simulink model "MSD2_RLS"  (R2019a)
settings: Solver=ode45  StartTime=t0  StopTime=tend  MaxStep=maxstep  RelTol=tol  AbsTol=tol
values from neighbouring files (symbols this model uses):
  d = 0.5    [SimMSD2_RLS.m]
  dx10 = 0    [SimMSD2_RLS.m]
  dx20 = 0    [SimMSD2_RLS.m]
  Fmag = 3    [SimMSD2_RLS.m]
  lambda = 0.99    [SimMSD2_RLS.m]
  P0 = 1e8 * eye(n_theta)    [SimMSD2_RLS.m]
  params_true = [m1 m2 k1 k2 c1 c2 b].'    [SimMSD2_RLS.m]
  T = 0.01    [SimMSD2_RLS.m]
  tend = 30    [SimMSD2_RLS.m]
  theta0 = genTheta(params0)    [SimMSD2_RLS.m]
  x10 = 0    [SimMSD2_RLS.m]
  x20 = x10    (= 0)    [SimMSD2_RLS.m]
  z0 = [x10 x20 dx10 dx20].'    [SimMSD2_RLS.m]
settings Model: Creator=bednarse  LastModifiedBy=bednarse

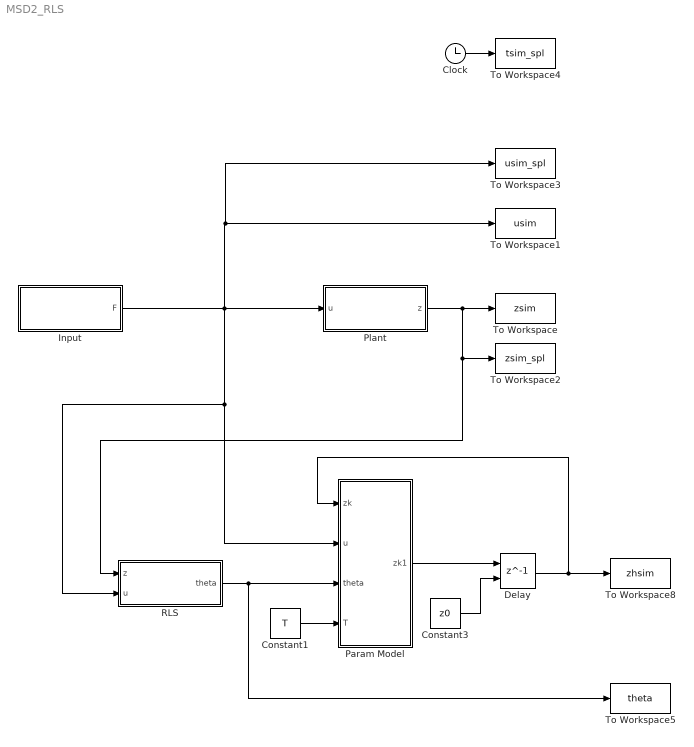
== system MSD2_RLS ==
  Clock : Clock
  Constant1 : Constant  Value=T
  Constant3 : Constant  Value=z0
  Delay : Delay  DelayLength=1  InitialConditionSource=Input port
      settings: InputPortMap=u0,p4
  Input : Subsystem
  Param Model : MATLAB Function  TreatAsAtomicUnit=on  SystemSampleTime=T
  Plant : Subsystem
  RLS : Subsystem
  To Workspace : ToWorkspace  VariableName=zsim  SampleTime=-1
  To Workspace1 : ToWorkspace  VariableName=usim  SampleTime=-1
  To Workspace2 : ToWorkspace  VariableName=zsim_spl  SampleTime=T
  To Workspace3 : ToWorkspace  VariableName=usim_spl  SampleTime=T
  To Workspace4 : ToWorkspace  VariableName=tsim_spl  SampleTime=T
  To Workspace5 : ToWorkspace  VariableName=theta  SampleTime=-1
  To Workspace8 : ToWorkspace  VariableName=zhsim  SampleTime=T
  wires:
  Plant/1(z) -> RLS/1(z), To Workspace2/1, To Workspace/1
  Clock/1 -> To Workspace4/1
  Param Model/1(zk1) -> Delay/1
  Constant1/1 -> Param Model/4(T)
  Constant3/1 -> Delay/2
  Delay/1 -> Param Model/1(zk), To Workspace8/1
  Input/1(F) -> Param Model/2(u), RLS/2(u), To Workspace3/1, To Workspace1/1, Plant/1(u)
  RLS/1(theta) -> To Workspace5/1, Param Model/3(theta)

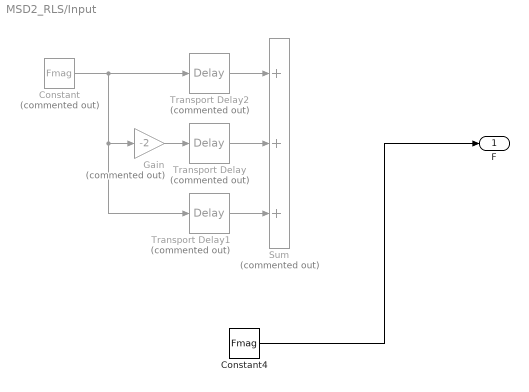
== system MSD2_RLS/Input ==
  Constant : Constant  Commented=on  Value=Fmag
  Constant4 : Constant  Value=Fmag
  Gain : Gain  Commented=on  Gain=-2
  Sum : Sum  Commented=on  Inputs=+++
  Transport Delay : TransportDelay  Commented=on  DelayTime=2*d  BufferSize=2048
  Transport Delay1 : TransportDelay  Commented=on  DelayTime=3*d  BufferSize=4096
  Transport Delay2 : TransportDelay  Commented=on  DelayTime=d
  F : Outport
  wires:
  Gain/1 -> Transport Delay/1
  Transport Delay1/1 -> Sum/3
  Transport Delay2/1 -> Sum/1
  Transport Delay/1 -> Sum/2
  Constant/1 -> Transport Delay1/1, Gain/1, Transport Delay2/1
  Constant4/1 -> F/1

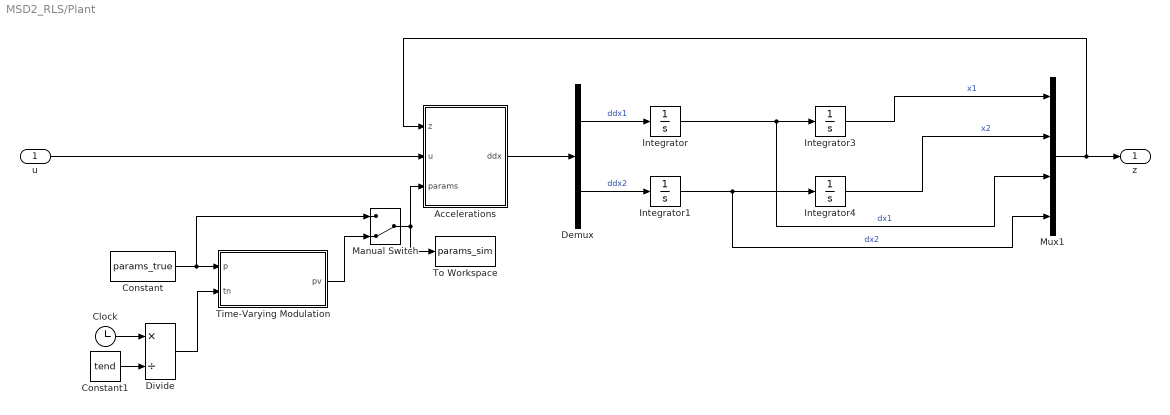
== system MSD2_RLS/Plant ==
  u : Inport
  Accelerations : MATLAB Function  TreatAsAtomicUnit=on
  Clock : Clock
  Constant : Constant  Value=params_true
  Constant1 : Constant  Value=tend
  Demux : Demux  Outputs=2
  Divide : Product  Inputs=*/
  Integrator : Integrator  InitialCondition=dx10
  Integrator1 : Integrator  InitialCondition=dx20
  Integrator3 : Integrator  InitialCondition=x10
  Integrator4 : Integrator  InitialCondition=x20
  Manual Switch : ManualSwitch  CurrentSetting=0
  Mux1 : Mux
  Time-Varying Modulation : MATLAB Function  TreatAsAtomicUnit=on
  To Workspace : ToWorkspace  VariableName=params_sim  SampleTime=-1
  z : Outport
  wires:
  Integrator3/1 -> Mux1/1  "x1"
  Integrator4/1 -> Mux1/2  "x2"
  Demux/2 -> Integrator1/1  "ddx2"
  Accelerations/1(ddx) -> Demux/1
  Demux/1 -> Integrator/1  "ddx1"
  Integrator/1 -> Mux1/3, Integrator3/1  "dx1"
  Integrator1/1 -> Mux1/4, Integrator4/1  "dx2"
  u/1 -> Accelerations/2(u)
  Mux1/1 -> Accelerations/1(z), z/1
  Clock/1 -> Divide/1
  Constant1/1 -> Divide/2
  Time-Varying Modulation/1(pv) -> Manual Switch/2
  Constant/1 -> Manual Switch/1, Time-Varying Modulation/1(p)
  Divide/1 -> Time-Varying Modulation/2(tn)
  Manual Switch/1 -> Accelerations/3(params), To Workspace/1

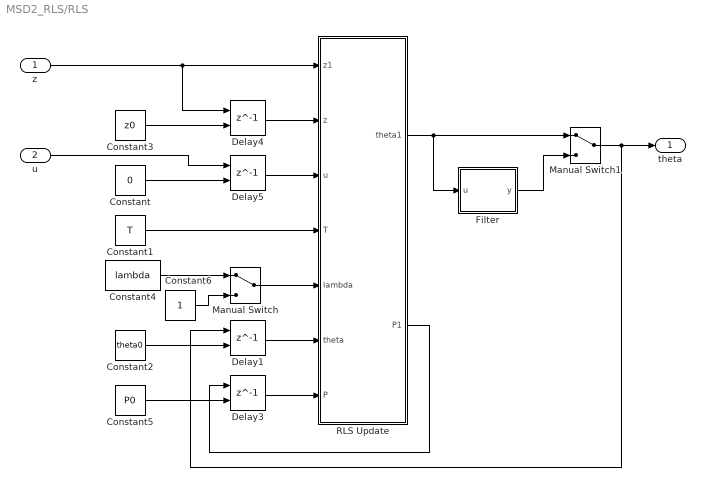
== system MSD2_RLS/RLS ==
  z : Inport
  u : Inport  Port=2
  Constant : Constant  Value=0
  Constant1 : Constant  Value=T
  Constant2 : Constant  Value=theta0
  Constant3 : Constant  Value=z0
  Constant4 : Constant  Value=lambda
  Constant5 : Constant  Value=P0
  Constant6 : Constant
  Delay{1,3..5} (4 alike) : Delay  DelayLength=1  InitialConditionSource=Input port
      settings: InputPortMap=u0,p4
  Filter : Subsystem
  Manual Switch : ManualSwitch
  Manual Switch1 : ManualSwitch
  RLS Update : MATLAB Function  TreatAsAtomicUnit=on  SystemSampleTime=T
  theta : Outport
  wires:
  Constant/1 -> Delay5/2
  Constant3/1 -> Delay4/2
  Constant5/1 -> Delay3/2
  Constant1/1 -> RLS Update/4(T)
  Constant2/1 -> Delay1/2
  Delay5/1 -> RLS Update/3(u)
  Delay4/1 -> RLS Update/2(z)
  Delay3/1 -> RLS Update/7(P)
  Delay1/1 -> RLS Update/6(theta)
  RLS Update/2(P1) -> Delay3/1
  u/1 -> Delay5/1
  z/1 -> Delay4/1, RLS Update/1(z1)
  Manual Switch/1 -> RLS Update/5(lambda)
  Constant6/1 -> Manual Switch/2
  Constant4/1 -> Manual Switch/1
  Manual Switch1/1 -> Delay1/1, theta/1
  RLS Update/1(theta1) -> Manual Switch1/1, Filter/1(u)
  Filter/1(y) -> Manual Switch1/2

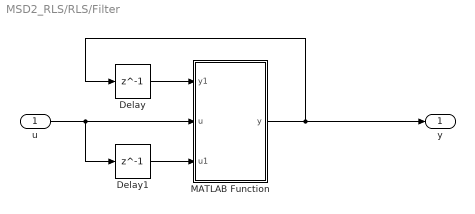
== system MSD2_RLS/RLS/Filter ==
  u : Inport
  Delay : Delay  DelayLength=1  InitialCondition=theta0
  Delay1 : Delay  DelayLength=1  InitialCondition=theta0
  MATLAB Function : MATLAB Function  TreatAsAtomicUnit=on  SystemSampleTime=T
  y : Outport
  wires:
  u/1 -> Delay1/1, MATLAB Function/2(u)
  Delay/1 -> MATLAB Function/1(y1)
  Delay1/1 -> MATLAB Function/3(u1)
  MATLAB Function/1(y) -> Delay/1, y/1

== matlab function MSD2_RLS/Plant/Time-Varying Modulation ==
  data: p input; pv output; tn input
function pv = vary_params(p, tn)

pv = p;
% pv(1) = p(1) + 0.1 * min(tn, 0.5) * 2;
if(tn >= 0.2)
    pv(1) = p(1) + 0.2;
end

== matlab function MSD2_RLS/Plant/Accelerations ==
  data: z input; u input; ddx output size=2; params input
function ddx  = msd2(z, u, params)

% Extract states
x1 = z(1);
x2 = z(2);
dx1 = z(3);
dx2 = z(4);

% Extract force inputs
F1 = u;

% Define system parameters
m1 = params(1);
m2 = params(2);
k1 = params(3);
k2 = params(4);
c1 = params(5);
c2 = params(6);
b = params(7);

% Form mass matrix
M = diag([m1 m2]);

% Form force vector
f = zeros(2, 1);
f(1) = k2*(x2-x1) + c2*(dx2-dx1) - k1*x1 - c1*dx1 - b*dx1 + F1;
f(2) = -k2*(x2-x1) - c2*(dx2-dx1) - b*dx2;

% Calculate accelerations
ddx = M \ f;

== matlab function MSD2_RLS/Param Model ==
  data: zk input; u input; zk1 output size=4; theta input; T input
function zk1 = fcn(zk, u, theta, T)

A = [zeros(2) eye(2); ...
    theta(1:4).'; ...
    theta(5:8).'];
B = [0 0 theta(9) 0].';

Ad = eye(4) + T * A;
Bd = T * B;

zk1 = Ad*zk + Bd*u;

== matlab function MSD2_RLS/RLS/Filter/MATLAB Function ==
  data: y1 input; u input; y output; u1 input
function y = lpf(y1, u, u1)

b1 = 0.04837;
b0 = 0.04679;
a0 = -0.9048;

b1 = 0.9;
b0 = 0.09995;
a0 = -4.54e-5;

y = b1*u + b0*u1 - a0*y1;

== matlab function MSD2_RLS/RLS/RLS Update ==
  data: z1 input; z input; u input; T input; lambda input; theta input; P input; theta1 output size=9; P1 output size=[9 9]
function[theta1, P1] =  msd2_rls(z1, z, u, T, lambda, theta, P)
    [phi, delta] = linParamFunc(z, u, T);
    
    KN = P * phi / (lambda * eye(4) + phi.' * P * phi);
    theta1 = theta + KN * (z1 - delta - phi.' * theta);
    P1 = (eye(9) - KN * phi.') * P / lambda;
end


function[phi, delta] = linParamFunc(z, u, T)
    phi = zeros(9, 4);
    phi(1:4, 3) = T * z;
    phi(9, 3) = T * u;
    phi(5:8, 4) = T * z;
    
    delta = [z(1)+T*z(3); ...
             z(2)+T*z(4); ...
                    z(3); ...
                    z(4)];
end
